simulink model "KTnTO"  (Simulink 10.0)
settings: Solver=ode45  StartTime=0.0  StopTime=0.02  MaxStep=0.0001  RelTol=1e-3  EnableMultiTasking=on
settings Model: Creator=mvcmv  LastModifiedBy=mvcmv
settings DataIOCC: LimitDataPoints=on  SignalLoggingSaveFormat=ModelDataLogs  SignalLoggingName=sigsOut
settings OptimizationCC: LifeSpan=auto
settings DebuggingCC: SaveWithParameterizedLinksMsg=none  SignalResolutionControl=TryResolveAllWithWarning  MultiTaskDSMMsg=warning  MultiTaskCondExecSysMsg=none  SFUnexpectedBacktrackingDiag=error  SFNoUnconditionalDefaultTransitionDiag=error  SFExecutionAtInitializationDiag=warning  ArithmeticOperatorsInVariantConditions=error
settings HardwareCC: TargetUnknown=on
settings SFSimCC: SimUseLocalCustomCode=on  CustomCodeUndefinedFunction=FilterOut
settings RTWCC: RTWUseLocalCustomCode=on
settings CodeAppCC: StateflowObjectComments=off
settings GRTTargetCC: TargetLangStandard=C99 (ISO)

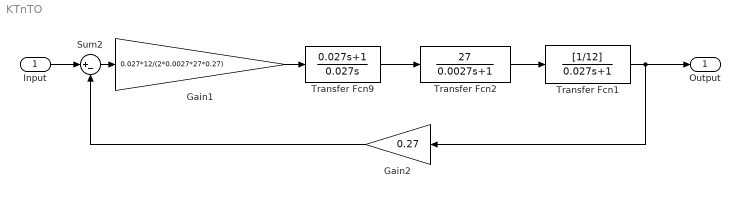
== system KTnTO ==
  Input : Inport
  Gain1 : Gain  Gain=0.027*12/(2*0.0027*27*0.27)  SaturateOnIntegerOverflow=on  OutDataTypeStr=Inherit: Same as input  ParamDataTypeStr=Inherit: Same as input
  Gain2 : Gain  Gain=0.27  SaturateOnIntegerOverflow=on  OutDataTypeStr=Inherit: Same as input  ParamDataTypeStr=Inherit: Same as input
  Sum2 : Sum  Inputs=|+-  SaturateOnIntegerOverflow=on
  Transfer Fcn1 : TransferFcn  Numerator=[1/12]  Denominator=[0.027 1]
  Transfer Fcn2 : TransferFcn  Numerator=[27]  Denominator=[0.0027 1]
  Transfer Fcn9 : TransferFcn  Numerator=[0.027 1]  Denominator=[0.027 0]
  Output : Outport
  wires:
  Transfer Fcn9/1 -> Transfer Fcn2/1
  Transfer Fcn2/1 -> Transfer Fcn1/1
  Gain1/1 -> Transfer Fcn9/1
  Sum2/1 -> Gain1/1
  Transfer Fcn1/1 -> Output/1, Gain2/1
  Gain2/1 -> Sum2/2
  Input/1 -> Sum2/1
